simulink model "Copy_of_generalized_energy_storage"  (R2021b)
settings: Solver=VariableStepAuto  StartTime=0.0  StopTime=3600  RelTol=1e-3
InitFcn:
  | %energy storage system
  | ess.Vdc_nom = 100;
  | ess.Vdc_0 = 100; %V
  | ess.Vdc_del = 50;
  | %ess.storageType = "bat"; %"sc" for supercapacitor, "bat" for battery
  | ess.storageType = "sc"; %"sc" for supercapacitor, "bat" for battery
  | 
  | ess.Ecap = 10; %total energy storage capacity, Wh
  | ess.isActive = 1;
  | ess.Cdc = 100e-6;
  | ess.kp_v = 0;
  | ess.ki_v = 0;
  | 
  | 
  | %determines the model parameters based on storage type, capacity, and
  | %nominal voltage
  | if ess.storageType == "bat"
  |     ess = ess_passive_bat_config(ess);
  | else %for now assume if not bat, do sc
  |     ess = ess_passive_sc_config(ess);
  | end
libraries: simulink x1
settings Model: Creator=jacksder  LastModifiedBy=Derek

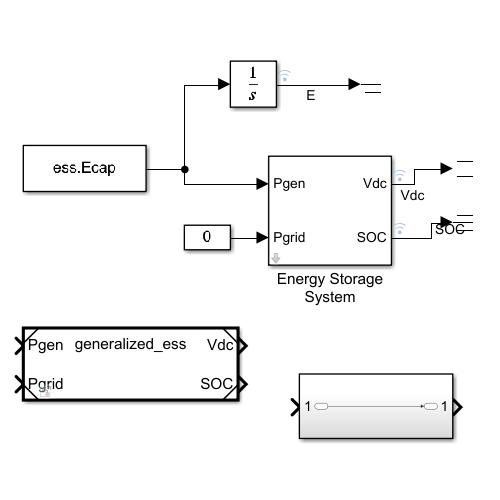
[thumbnail: Simulink's stored preview of the top-level diagram]
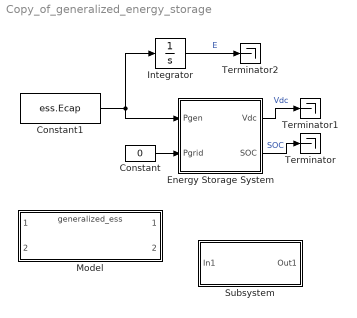
== system Copy_of_generalized_energy_storage ==
  Constant : Constant  Value=0
  Constant1 : Constant  Value=ess.Ecap
  Energy Storage System : Subsystem  mask{ess=ess}
      mask prompts: ess "ESS data structure:"
      mask DialogControl DescTextVar_copy Prompt: Uses a generalized energy storage model.
      mask DialogControl ParamGroupVar Prompt: Energy Storage System Parameters
  Integrator : Integrator
  Model : ModelReference  ModelNameDialog=generalized_ess  SimulationMode=Normal  ModelReferenceVersion=1.2
  Subsystem : Subsystem
  Terminator : Terminator
  Terminator1 : Terminator
  Terminator2 : Terminator
  wires:
  Constant/1 -> Energy Storage System/2(Pgrid)
  Constant1/1 -> Integrator/1, Energy Storage System/1(Pgen)
  Energy Storage System/2(SOC) -> Terminator/1  "SOC"
  Energy Storage System/1(Vdc) -> Terminator1/1  "Vdc"
  Integrator/1 -> Terminator2/1  "E"

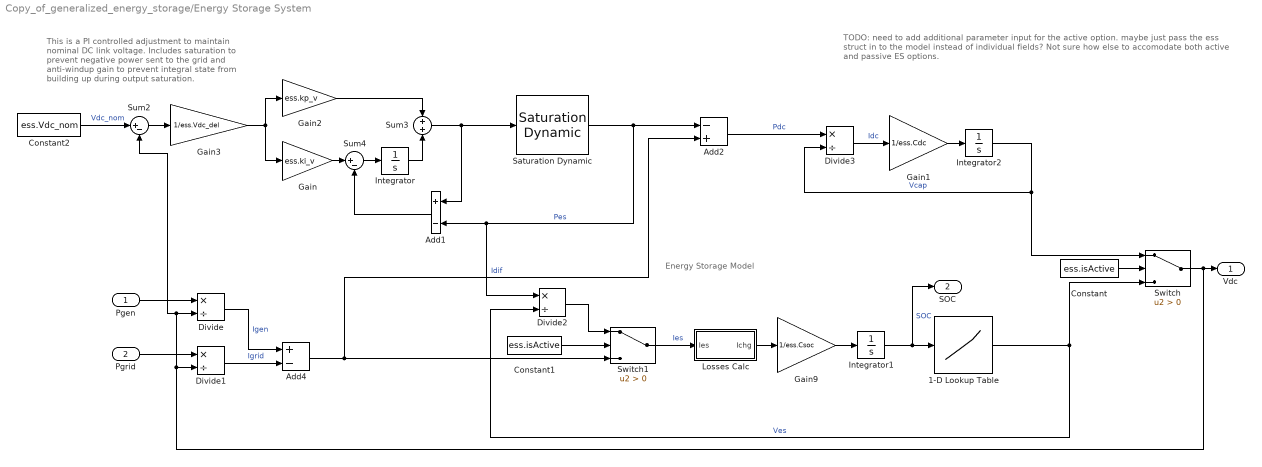
== system Copy_of_generalized_energy_storage/Energy Storage System ==
  note: TODO: need to add additional parameter input for the active option. maybe just pass the ess struct in to the model instead of individual fields? Not sure how else to accomodate both active and passive ES options.
  note: Energy Storage Model
  note: This is a PI controlled adjustment to maintain nominal DC link voltage. Includes saturation to prevent negative power sent to the grid and anti-windup gain to prevent integral state from building up during output saturation.
  Pgen : Inport
  Pgrid : Inport  Port=2
  1-D Lookup Table : Lookup_n-D  NumberOfTableDimensions=1  BreakpointsForDimension1=ess.SOC_LUT  Table=ess.Voc_LUT  InternalRulePriority=Speed  RndMeth=Simplest  InputSameDT=on
  Add1 : Sum  Inputs=+-
  Add2 : Sum  Inputs=-+
  Add4 : Sum  Inputs=+-
  Constant : Constant  Value=ess.isActive
  Constant1 : Constant  Value=ess.isActive
  Constant2 : Constant  Value=ess.Vdc_nom
  Divide{,1..3} (4 alike) : Product  Inputs=*/
  Gain : Gain  Gain=ess.ki_v
  Gain1 : Gain  Gain=1/ess.Cdc
  Gain2 : Gain  Gain=ess.kp_v
  Gain3 : Gain  Gain=1/ess.Vdc_del
  Gain9 : Gain  Gain=1/ess.Csoc
  Integrator : Integrator
  Integrator1 : Integrator  InitialCondition=ess.SOC_0
  Integrator2 : Integrator  InitialCondition=ess.Vdc_0
  Losses Calc : Subsystem
  Saturation Dynamic : simulink/Discontinuities/Saturation Dynamic  OutMin=[]  OutMax=[]  OutDataTypeStr=Inherit: Same as second input  OutDataType=fixdt(1, 16)  OutScaling=2^-10  DoSatur=off
  Sum2 : Sum  Inputs=|+-
  Sum3 : Sum
  Sum4 : Sum  Inputs=|+-
  Switch : Switch  Criteria=u2 > Threshold
  Switch1 : Switch  Criteria=u2 > Threshold
  Vdc : Outport
  SOC : Outport  Port=2
  wires:
  Pgrid/1 -> Divide1/1
  Pgen/1 -> Divide/1
  Divide1/1 -> Add4/2  "Igrid"
  Gain9/1 -> Integrator1/1
  Divide/1 -> Add4/1  "Igen"
  Integrator1/1 -> SOC/1, 1-D Lookup Table/1  "SOC"
  Switch1/1 -> Losses Calc/1(Ies)  "Ies"
  Losses Calc/1(Ichg) -> Gain9/1
  Switch/1 -> Sum2/2, Divide/2, Divide1/2, Vdc/1
  Gain1/1 -> Integrator2/1
  Divide3/1 -> Gain1/1  "Idc"
  Constant/1 -> Switch/2
  Integrator2/1 -> Switch/1, Divide3/2  "Vcap"
  1-D Lookup Table/1 -> Divide2/2, Switch/3  "Ves"
  Constant1/1 -> Switch1/2
  Add4/1 -> Add2/2, Switch1/3  "Idif"
  Gain/1 -> Sum4/1
  Add1/1 -> Sum4/2
  Integrator/1 -> Sum3/2
  Sum4/1 -> Integrator/1
  Saturation Dynamic/1 -> Divide2/1, Add1/2, Add2/1  "Pes"
  Gain3/1 -> Gain2/1, Gain/1
  Gain2/1 -> Sum3/1
  Sum2/1 -> Gain3/1
  Sum3/1 -> Add1/1, Saturation Dynamic/2
  Constant2/1 -> Sum2/1  "Vdc_nom"
  Divide2/1 -> Switch1/1
  Add2/1 -> Divide3/1  "Pdc"

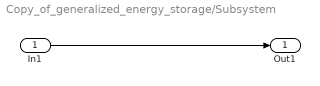
== system Copy_of_generalized_energy_storage/Subsystem ==
  In1 : Inport
  Out1 : Outport
  wires:
  In1/1 -> Out1/1

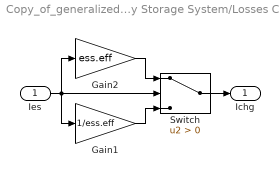
== system Copy_of_generalized_energy_storage/Energy Storage System/Losses Calc ==
  Ies : Inport
  Gain1 : Gain  Gain=1/ess.eff
  Gain2 : Gain  Gain=ess.eff
  Switch : Switch  Criteria=u2 > Threshold
  Ichg : Outport
  wires:
  Ies/1 -> Gain1/1, Gain2/1, Switch/2
  Switch/1 -> Ichg/1
  Gain2/1 -> Switch/1
  Gain1/1 -> Switch/3
